simulink library "mcs_new"  (Simulink 8.1)
settings: Solver=ode1  StartTime=0.0  StopTime=Inf  FixedStep=0.001  RelTol=1e-3
PostLoadFcn:
  | , if any(exist('dsrtsu_mdlpostloadfcn', 'file') == [2, 3, 6]), try dsrtsu_mdlpostloadfcn('Execute', bdroot); catch fprintf('Error in PostLoadFcn (dsrtsu_mdlpostloadfcn) for model "%s":\n %s\n', bdroot, lasterr); end, end,
libraries: vpc x1, vpc_new x1, mct x1, mct_new x1, sdc x1, tty x1, tdc x1, ipb x1, vip x1
settings Model: DSRTSU_INTERNAL_RTI_VER=450  DSRTSU_INTERNAL_RTI_TYPE=rti1401  RTICANMMDATA=struct('GeneralSetupData',struct('modelroot','D:\PROJECTS\HAITEC\TAIWAN_HAITEC_SVN\trunk\AdasDragon\software\sw_development\arch\app\ifo','generalsettings',struct('filesettings',struct('destfolder',struct('Name','RTICANMM_FILES','Check',1),'buildfolder',struct('Name','.','Check',1),'AbsDestfolder',struct('Name','D:\PROJECTS\HAITEC\TAIWAN_HAITEC_SVN\trunk\AdasDragon\software\sw_development\arch\app\ifo\RTICANMM_FILES'),'AbsBuildfolder',struct('Name','D:\PROJECTS\HAITEC\TAIWAN_HAITEC_SVN\trunk\AdasDragon\software\sw_development\arch\app\ifo'))),'options',struct('addpaths',1,'rmpaths',1,'addtrcexclusion',logical(1),'cannavigator',struct('checkmonitoring',0),'show_usrtrc',0,'use_usrtrc',0),'advanced',struct('options',[1 1 1 1 1 1 1 1 1 1 1 1 1 1 1 1 1 1 1 1 1 1 1 1 1 1 1 1 1 1 1 1 1 1 1 1 1 1 1 1 1 1 1 1 1 1 1 1 1 1 1 1 1 1 1 1 1 1 1 1 1 1 1 1 1 1 1 1 1 1 1 1 1 1 1 1 1 1 1 1 1 1 1 1 1 1 1 1 1 1 1 1 1 1 1 1 1 1 1 1]),'MPSetup',{{}},'modelname','mcs','block','mcs'))  DSRTSU_INTERNAL_RTIFPGA=40  Creator=tescamilla  LastModifiedBy=tescamilla

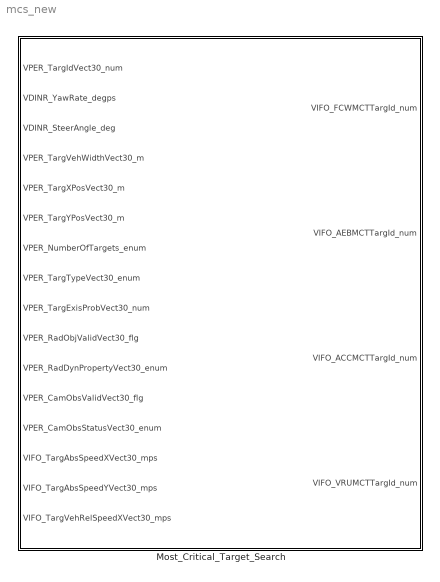
== system mcs_new ==
  Most_Critical_Target_Search : Subsystem

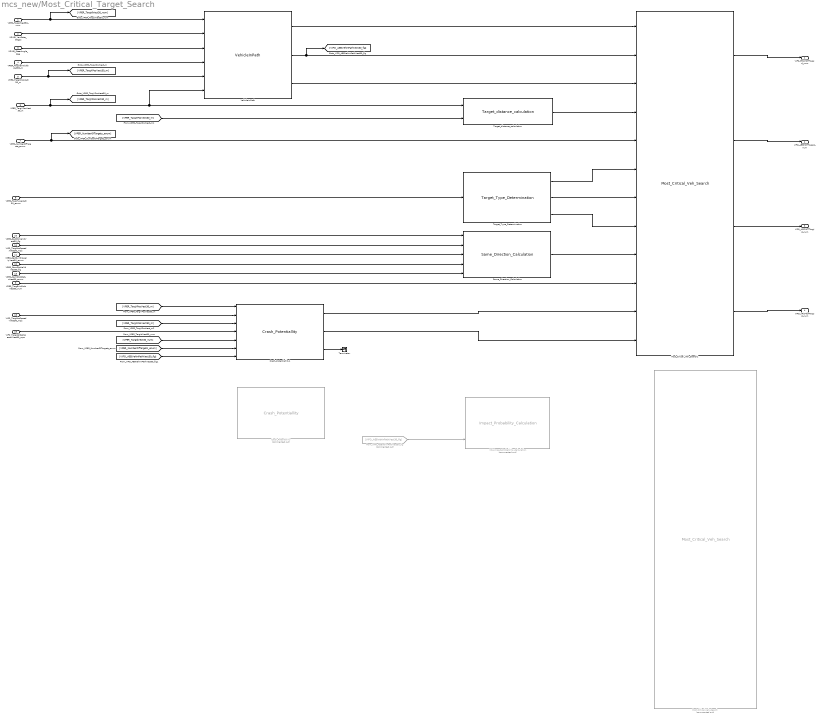
== system mcs_new/Most_Critical_Target_Search ==
  VPER_TargIdVect30_num : Inport
  VDINR_YawRate_degps : Inport  Port=2
  VDINR_SteerAngle_deg : Inport  Port=3
  VPER_TargVehWidthVect30_m : Inport  Port=4
  VPER_TargXPosVect30_m : Inport  Port=5
  VPER_TargYPosVect30_m : Inport  Port=6
  VPER_NumberOfTargets_enum : Inport  Port=7
  VPER_TargTypeVect30_enum : Inport  Port=8
  VPER_TargExisProbVect30_num : Inport  Port=9
  VPER_RadObjValidVect30_flg : Inport  Port=10
  VPER_RadDynPropertyVect30_enum : Inport  Port=11
  VPER_CamObsValidVect30_flg : Inport  Port=12
  VPER_CamObsStatusVect30_enum : Inport  Port=13
  VIFO_TargAbsSpeedXVect30_mps : Inport  Port=14
  VIFO_TargAbsSpeedYVect30_mps : Inport  Port=15
  VIFO_TargVehRelSpeedXVect30_mps : Inport  Port=16
  Crash_Potentiallity : vpc/Crash_Potentiallity  Commented=on
  Crash_Potentiallity1 : vpc_new/Crash_Potentiallity
  From_VIFO_AEBVehInPathVect30_flg : From  Commented=on  GotoTag=VIFO_AEBVehInPathVect30_flg
  Most_Critical_Veh_Search : mct/Most_Critical_Veh_Search  Commented=on
  Most_Critical_Veh_Search1 : mct_new/Most_Critical_Veh_Search
  Same_Direction_Calculation : sdc/Same_Direction_Calculation
  Target_Type_Determination : tty/Target_Type_Determination
  Target_distance_calculation : tdc/Target_distance_calculation
  Terminator : Terminator
  VRU_Impact_Probability_Calculation : ipb/Impact_Probability_Calculation  Commented=on
  VehicleInPath : vip/VehicleInPath
  VIFO_FCWMCTTargId_num : Outport
  VIFO_AEBMCTTargId_num : Outport  Port=2
  VIFO_ACCMCTTargId_num : Outport  Port=3
  VIFO_VRUMCTTargId_num : Outport  Port=4
  wires:
  Target_Type_Determination/1 -> Most_Critical_Veh_Search1/6
  Target_Type_Determination/2 -> Most_Critical_Veh_Search1/7
  VehicleInPath/3 -> Most_Critical_Veh_Search1/3
  Most_Critical_Veh_Search1/3 -> VIFO_ACCMCTTargId_num/1
  VPER_TargYPosVect30_m/1 -> [VPER_TargYPosVect30_m], VehicleInPath/6, Target_distance_calculation/1
  VPER_TargVehWidthVect30_m/1 -> VehicleInPath/4
  VPER_TargXPosVect30_m/1 -> VehicleInPath/5, [VPER_TargXPosVect30_m]
  VehicleInPath/1 -> Most_Critical_Veh_Search1/1
  VehicleInPath/2 -> [VIFO_AEBVehInPathVect30_flg], Most_Critical_Veh_Search1/2
  Target_distance_calculation/1 -> Most_Critical_Veh_Search1/4
  Same_Direction_Calculation/1 -> Most_Critical_Veh_Search1/9
  VPER_TargTypeVect30_enum/1 -> Target_Type_Determination/1
  VDINR_YawRate_degps/1 -> VehicleInPath/2
  [VPER_TargXPosVect30_m] -> Target_distance_calculation/2
  VDINR_SteerAngle_deg/1 -> VehicleInPath/3
  VPER_NumberOfTargets_enum/1 -> [VPER_NumberOfTargets_enum], Most_Critical_Veh_Search1/5
  Most_Critical_Veh_Search1/2 -> VIFO_AEBMCTTargId_num/1
  Most_Critical_Veh_Search1/1 -> VIFO_FCWMCTTargId_num/1
  VIFO_TargAbsSpeedXVect30_mps/1 -> Same_Direction_Calculation/2
  VPER_TargExisProbVect30_num/1 -> Most_Critical_Veh_Search1/10
  VPER_TargIdVect30_num/1 -> [VPER_TargIdVect30_num], VehicleInPath/1
  VPER_RadDynPropertyVect30_enum/1 -> Same_Direction_Calculation/3
  VPER_CamObsValidVect30_flg/1 -> Same_Direction_Calculation/4
  VPER_CamObsStatusVect30_enum/1 -> Same_Direction_Calculation/5
  VPER_RadObjValidVect30_flg/1 -> Same_Direction_Calculation/1
  Target_Type_Determination/3 -> Most_Critical_Veh_Search1/8
  Crash_Potentiallity1/3 -> Terminator/1
  Crash_Potentiallity1/2 -> Most_Critical_Veh_Search1/12
  Crash_Potentiallity1/1 -> Most_Critical_Veh_Search1/11
  Most_Critical_Veh_Search1/4 -> VIFO_VRUMCTTargId_num/1
  [VPER_TargXPosVect30_m] -> Crash_Potentiallity1/3
  [VPER_TargYPosVect30_m] -> Crash_Potentiallity1/1
  VIFO_TargAbsSpeedYVect30_mps/1 -> Crash_Potentiallity1/2
  VIFO_TargVehRelSpeedXVect30_mps/1 -> Crash_Potentiallity1/4
  From_VIFO_AEBVehInPathVect30_flg/1 -> VRU_Impact_Probability_Calculation/3
  [VPER_TargIdVect30_num] -> Crash_Potentiallity1/5
  [VPER_NumberOfTargets_enum] -> Crash_Potentiallity1/6
  [VIFO_AEBVehInPathVect30_flg] -> Crash_Potentiallity1/7
